simulink model "model"  (R2018a)
settings: Solver=FixedStepAuto  StartTime=0.0  StopTime=inf  FixedStep=0.1  MaxStep=0.1  MinStep=0.001  RelTol=1e-3
libraries: vrlib x19, simulink x15
(part 2 of 2)

== system model/opponent_scout/rand_pos_gen ==
  x_max : Inport
  y_max : Inport  Port=2
  x : Inport  Port=3
  y : Inport  Port=4
  Enable : EnablePort
  Constant : Constant  Value=2
  IC : InitialCondition  Value=0
  Less Than : RelationalOperator  Operator=<  OutDataTypeStr=boolean  RndMeth=Simplest
  Memory : Memory
  Terminator : Terminator
  get_vector : Subsystem
  rand_position_gen : Subsystem
  new_x : Outport
  new_y : Outport  Port=2
  wires:
  get_vector/2(angle) -> Terminator/1
  y/1 -> get_vector/4(y1)
  Less Than/1 -> Memory/1
  Memory/1 -> rand_position_gen/Trigger
  x_max/1 -> rand_position_gen/1(x_max)
  x/1 -> get_vector/2(x1)
  rand_position_gen/1(x_out) -> new_x/1, get_vector/1(x2)
  get_vector/1(distance) -> IC/1
  rand_position_gen/2(y_out) -> new_y/1, get_vector/3(y2)
  y_max/1 -> rand_position_gen/2(y_max)
  Constant/1 -> Less Than/2
  IC/1 -> Less Than/1

== system model/scout/est_theta ==
  r : Inport
  l : Inport  Port=2
  ur : Inport  Port=3
  ul : Inport  Port=4
  theta_0 : Inport  Port=5
  Divide : Product  Inputs=**/
  Integrator : Integrator  InitialConditionSource=external
  Minus : Sum  Inputs=+-
  theta : Outport
  wires:
  theta_0/1 -> Integrator/2
  ur/1 -> Minus/2
  l/1 -> Divide/3
  Minus/1 -> Divide/2
  r/1 -> Divide/1
  ul/1 -> Minus/1
  Integrator/1 -> theta/1
  Divide/1 -> Integrator/1

== system model/scout/est_x ==
  r : Inport
  theta : Inport  Port=2
  ul : Inport  Port=3
  ur : Inport  Port=4
  x0 : Inport  Port=5
  Add : Sum
  Cos : Trigonometry  Operator=cos
  Gain : Gain  Gain=1/2
  Integrator : Integrator  InitialConditionSource=external
  Multiply : Product  Inputs=3
  x : Outport
  wires:
  r/1 -> Multiply/1
  ur/1 -> Add/2
  Add/1 -> Multiply/2
  theta/1 -> Cos/1
  Cos/1 -> Multiply/3
  Integrator/1 -> x/1
  Multiply/1 -> Gain/1
  ul/1 -> Add/1
  Gain/1 -> Integrator/1
  x0/1 -> Integrator/2

== system model/scout/est_y ==
  r : Inport
  theta : Inport  Port=2
  ul : Inport  Port=3
  ur : Inport  Port=4
  y0 : Inport  Port=5
  ref_y : Inport  Port=6
  Add : Sum
  Cos : Trigonometry
  Detect Change : simulink/Logic and Bit Operations/Detect Change  vinit=0  OutDataTypeStr=boolean
  Gain : Gain  Gain=1/2
  Integrator : Integrator  ExternalReset=rising  InitialConditionSource=external
  Multiply : Product  Inputs=3
  Switch : Switch  Criteria=u2 > Threshold
  y : Outport
  wires:
  r/1 -> Multiply/1
  ur/1 -> Add/2
  Add/1 -> Multiply/2
  theta/1 -> Cos/1
  Cos/1 -> Multiply/3
  Integrator/1 -> y/1
  Multiply/1 -> Gain/1
  ul/1 -> Add/1
  Gain/1 -> Integrator/1
  y0/1 -> Switch/3
  ref_y/1 -> Switch/1, Detect Change/1
  Detect Change/1 -> Switch/2, Integrator/2
  Switch/1 -> Integrator/3

== system model/scout/get_vector_to_destination ==
  x2 : Inport
  x1 : Inport  Port=2
  y2 : Inport  Port=3
  y1 : Inport  Port=4
  Add : Sum
  Atan2 : Trigonometry  Operator=atan2
  Minus : Sum  Inputs=+-
  Minus1 : Sum  Inputs=+-
  Sqrt : Sqrt  SaturateOnIntegerOverflow=on
  Square : Math  Operator=square  SaturateOnIntegerOverflow=on
  Square1 : Math  Operator=square  SaturateOnIntegerOverflow=on
  distance : Outport
  angle : Outport  Port=2
  wires:
  Minus/1 -> Atan2/2, Square1/1
  y1/1 -> Minus1/2
  Square/1 -> Add/2
  Minus1/1 -> Atan2/1, Square/1
  Add/1 -> Sqrt/1
  Square1/1 -> Add/1
  x1/1 -> Minus/2
  x2/1 -> Minus/1
  Sqrt/1 -> distance/1
  y2/1 -> Minus1/1
  Atan2/1 -> angle/1

== system model/scout/pid ==
  ref_out : Inport
  act_out : Inport  Port=2
  Kp : Inport  Port=3
  Ki : Inport  Port=4
  Kd : Inport  Port=5
  Enable : EnablePort  StatesWhenEnabling=reset
  Discrete Derivative : simulink/Discrete/Discrete Derivative  gainval=1.0  ICPrevScaledInput=0.0  OutMin=[]  OutMax=[]  OutDataType=fixdt(1, 16)  OutScaling=2^-10  DoSatur=off
  Integrator : Integrator
  Multiply : Product
  Multiply1 : Product
  Multiply2 : Product
  Sum : Sum  Inputs=|+-
  Sum1 : Sum  Inputs=+++
  new_out : Outport
  wires:
  act_out/1 -> Sum/2
  Ki/1 -> Multiply1/2
  Multiply/1 -> Sum1/1
  Kd/1 -> Multiply2/2
  Sum/1 -> Multiply/1, Integrator/1, Discrete Derivative/1
  Kp/1 -> Multiply/2
  ref_out/1 -> Sum/1
  Integrator/1 -> Multiply1/1
  Multiply1/1 -> Sum1/2
  Multiply2/1 -> Sum1/3
  Sum1/1 -> new_out/1
  Discrete Derivative/1 -> Multiply2/1

== system model/scout/pid1 ==
  ref_out : Inport
  act_out : Inport  Port=2
  Kp : Inport  Port=3
  Ki : Inport  Port=4
  Kd : Inport  Port=5
  Enable : EnablePort  StatesWhenEnabling=reset
  Discrete Derivative : simulink/Discrete/Discrete Derivative  gainval=1.0  ICPrevScaledInput=0.0  OutMin=[]  OutMax=[]  OutDataType=fixdt(1, 16)  OutScaling=2^-10  DoSatur=off
  Integrator : Integrator
  Multiply : Product
  Multiply1 : Product
  Multiply2 : Product
  Sum : Sum  Inputs=|+-
  Sum1 : Sum  Inputs=+++
  new_out : Outport
  wires:
  Discrete Derivative/1 -> Multiply2/1
  Sum1/1 -> new_out/1
  Multiply2/1 -> Sum1/3
  Multiply1/1 -> Sum1/2
  Integrator/1 -> Multiply1/1
  ref_out/1 -> Sum/1
  Kp/1 -> Multiply/2
  Sum/1 -> Discrete Derivative/1, Integrator/1, Multiply/1
  Kd/1 -> Multiply2/2
  Multiply/1 -> Sum1/1
  Ki/1 -> Multiply1/2
  act_out/1 -> Sum/2

== system model/scout/rand_pos_gen ==
  x_max : Inport
  y_max : Inport  Port=2
  x : Inport  Port=3
  y : Inport  Port=4
  Constant : Constant  Value=2
  Less Than : RelationalOperator  Operator=<  OutDataTypeStr=boolean  RndMeth=Simplest
  Memory : Memory
  Terminator : Terminator
  get_vector : Subsystem
  rand_position_gen : Subsystem
  new_x : Outport
  new_y : Outport  Port=2
  wires:
  get_vector/2(angle) -> Terminator/1
  y/1 -> get_vector/4(y1)
  Less Than/1 -> Memory/1
  Memory/1 -> rand_position_gen/Trigger
  x_max/1 -> rand_position_gen/1(x_max)
  x/1 -> get_vector/2(x1)
  rand_position_gen/1(x_out) -> new_x/1, get_vector/1(x2)
  get_vector/1(distance) -> Less Than/1
  rand_position_gen/2(y_out) -> new_y/1, get_vector/3(y2)
  y_max/1 -> rand_position_gen/2(y_max)
  Constant/1 -> Less Than/2

== system model/scout/real_theta ==
  r : Inport
  l : Inport  Port=2
  ur : Inport  Port=3
  ul : Inport  Port=4
  theta_0 : Inport  Port=5
  Divide : Product  Inputs=**/
  Integrator : Integrator  InitialConditionSource=external
  Minus : Sum  Inputs=+-
  theta : Outport
  wires:
  theta_0/1 -> Integrator/2
  ur/1 -> Minus/2
  l/1 -> Divide/3
  Minus/1 -> Divide/2
  r/1 -> Divide/1
  ul/1 -> Minus/1
  Integrator/1 -> theta/1
  Divide/1 -> Integrator/1

== system model/scout/real_x ==
  r : Inport
  theta : Inport  Port=2
  ul : Inport  Port=3
  ur : Inport  Port=4
  x0 : Inport  Port=5
  dx_in : Inport  Port=6
  Add : Sum
  Cos : Trigonometry  Operator=cos
  Gain : Gain  Gain=1/2
  Gain1 : Gain  Gain=1.1
  Integrator : Integrator  InitialConditionSource=external
  Multiply : Product  Inputs=3
  Switch : Switch  Criteria=u2 ~= 0
  x : Outport
  dx : Outport  Port=2
  wires:
  r/1 -> Multiply/1
  ur/1 -> Add/2
  Add/1 -> Multiply/2
  theta/1 -> Cos/1
  Cos/1 -> Multiply/3
  Integrator/1 -> x/1
  Multiply/1 -> Gain/1
  ul/1 -> Add/1
  Gain/1 -> Switch/3, dx/1
  x0/1 -> Integrator/2
  dx_in/1 -> Switch/2, Gain1/1
  Switch/1 -> Integrator/1
  Gain1/1 -> Switch/1

== system model/scout/real_y ==
  r : Inport
  theta : Inport  Port=2
  ul : Inport  Port=3
  ur : Inport  Port=4
  y0 : Inport  Port=5
  dy_in : Inport  Port=6
  Add : Sum
  Cos : Trigonometry
  Gain : Gain  Gain=1/2
  Gain1 : Gain  Gain=1.1
  Integrator : Integrator  InitialConditionSource=external
  Multiply : Product  Inputs=3
  Switch : Switch  Criteria=u2 ~= 0
  y : Outport
  dy : Outport  Port=2
  wires:
  r/1 -> Multiply/1
  ur/1 -> Add/2
  Add/1 -> Multiply/2
  theta/1 -> Cos/1
  Cos/1 -> Multiply/3
  Integrator/1 -> y/1
  Multiply/1 -> Gain/1
  ul/1 -> Add/1
  Gain/1 -> Switch/3, dy/1
  y0/1 -> Integrator/2
  dy_in/1 -> Gain1/1, Switch/2
  Switch/1 -> Integrator/1
  Gain1/1 -> Switch/1

== system model/light_spot/rand_pos_gen/get_vector ==
  x2 : Inport
  x1 : Inport  Port=2
  y2 : Inport  Port=3
  y1 : Inport  Port=4
  Add : Sum
  Atan2 : Trigonometry  Operator=atan2
  Minus : Sum  Inputs=+-
  Minus1 : Sum  Inputs=+-
  Sqrt : Sqrt  SaturateOnIntegerOverflow=on
  Square : Math  Operator=square  SaturateOnIntegerOverflow=on
  Square1 : Math  Operator=square  SaturateOnIntegerOverflow=on
  distance : Outport
  angle : Outport  Port=2
  wires:
  Minus/1 -> Atan2/2, Square1/1
  y1/1 -> Minus1/2
  Square/1 -> Add/2
  Minus1/1 -> Atan2/1, Square/1
  Add/1 -> Sqrt/1
  Square1/1 -> Add/1
  x1/1 -> Minus/2
  x2/1 -> Minus/1
  Sqrt/1 -> distance/1
  y2/1 -> Minus1/1
  Atan2/1 -> angle/1

== system model/light_spot/rand_pos_gen/rand_position_gen ==
  x_max : Inport
  y_max : Inport  Port=2
  Trigger : TriggerPort  VariantControl=Variant  PortDimensions=1
  Multiply : Product
  Multiply1 : Product
  x : UniformRandomNumber  Minimum=0  Seed=172
  y : UniformRandomNumber  Minimum=0  Seed=22
  x_out : Outport
  y_out : Outport  Port=2
  wires:
  y_max/1 -> Multiply/1
  x/1 -> Multiply1/2
  y/1 -> Multiply/2
  x_max/1 -> Multiply1/1
  Multiply1/1 -> x_out/1
  Multiply/1 -> y_out/1

== system model/opponent_collector/rand_pos_gen/get_vector ==
  x2 : Inport
  x1 : Inport  Port=2
  y2 : Inport  Port=3
  y1 : Inport  Port=4
  Add : Sum
  Atan2 : Trigonometry  Operator=atan2
  Minus : Sum  Inputs=+-
  Minus1 : Sum  Inputs=+-
  Sqrt : Sqrt  SaturateOnIntegerOverflow=on
  Square : Math  Operator=square  SaturateOnIntegerOverflow=on
  Square1 : Math  Operator=square  SaturateOnIntegerOverflow=on
  distance : Outport
  angle : Outport  Port=2
  wires:
  Minus/1 -> Atan2/2, Square1/1
  y1/1 -> Minus1/2
  Square/1 -> Add/2
  Minus1/1 -> Atan2/1, Square/1
  Add/1 -> Sqrt/1
  Square1/1 -> Add/1
  x1/1 -> Minus/2
  x2/1 -> Minus/1
  Sqrt/1 -> distance/1
  y2/1 -> Minus1/1
  Atan2/1 -> angle/1

== system model/opponent_collector/rand_pos_gen/rand_position_gen ==
  x_max : Inport
  y_max : Inport  Port=2
  Trigger : TriggerPort  VariantControl=Variant  PortDimensions=1
  Multiply : Product
  Multiply1 : Product
  x : UniformRandomNumber  Minimum=0  Seed=1
  y : UniformRandomNumber  Minimum=0  Seed=110
  x_out : Outport
  y_out : Outport  Port=2
  wires:
  y_max/1 -> Multiply/1
  x/1 -> Multiply1/2
  y/1 -> Multiply/2
  x_max/1 -> Multiply1/1
  Multiply1/1 -> x_out/1
  Multiply/1 -> y_out/1

== system model/opponent_scout/rand_pos_gen/get_vector ==
  x2 : Inport
  x1 : Inport  Port=2
  y2 : Inport  Port=3
  y1 : Inport  Port=4
  Add : Sum
  Atan2 : Trigonometry  Operator=atan2
  Minus : Sum  Inputs=+-
  Minus1 : Sum  Inputs=+-
  Sqrt : Sqrt  SaturateOnIntegerOverflow=on
  Square : Math  Operator=square  SaturateOnIntegerOverflow=on
  Square1 : Math  Operator=square  SaturateOnIntegerOverflow=on
  distance : Outport
  angle : Outport  Port=2
  wires:
  Minus/1 -> Atan2/2, Square1/1
  y1/1 -> Minus1/2
  Square/1 -> Add/2
  Minus1/1 -> Atan2/1, Square/1
  Add/1 -> Sqrt/1
  Square1/1 -> Add/1
  x1/1 -> Minus/2
  x2/1 -> Minus/1
  Sqrt/1 -> distance/1
  y2/1 -> Minus1/1
  Atan2/1 -> angle/1

== system model/opponent_scout/rand_pos_gen/rand_position_gen ==
  x_max : Inport
  y_max : Inport  Port=2
  Trigger : TriggerPort  VariantControl=Variant  PortDimensions=1
  Multiply : Product
  Multiply1 : Product
  x : UniformRandomNumber  Minimum=0  Seed=213
  y : UniformRandomNumber  Minimum=0  Seed=130
  x_out : Outport
  y_out : Outport  Port=2
  wires:
  y_max/1 -> Multiply/1
  x/1 -> Multiply1/2
  y/1 -> Multiply/2
  x_max/1 -> Multiply1/1
  Multiply1/1 -> x_out/1
  Multiply/1 -> y_out/1

== system model/scout/rand_pos_gen/get_vector ==
  x2 : Inport
  x1 : Inport  Port=2
  y2 : Inport  Port=3
  y1 : Inport  Port=4
  Add : Sum
  Atan2 : Trigonometry  Operator=atan2
  Minus : Sum  Inputs=+-
  Minus1 : Sum  Inputs=+-
  Sqrt : Sqrt  SaturateOnIntegerOverflow=on
  Square : Math  Operator=square  SaturateOnIntegerOverflow=on
  Square1 : Math  Operator=square  SaturateOnIntegerOverflow=on
  distance : Outport
  angle : Outport  Port=2
  wires:
  Minus/1 -> Atan2/2, Square1/1
  y1/1 -> Minus1/2
  Square/1 -> Add/2
  Minus1/1 -> Atan2/1, Square/1
  Add/1 -> Sqrt/1
  Square1/1 -> Add/1
  x1/1 -> Minus/2
  x2/1 -> Minus/1
  Sqrt/1 -> distance/1
  y2/1 -> Minus1/1
  Atan2/1 -> angle/1

== system model/scout/rand_pos_gen/rand_position_gen ==
  x_max : Inport
  y_max : Inport  Port=2
  Trigger : TriggerPort  VariantControl=Variant  PortDimensions=1
  Multiply : Product
  Multiply1 : Product
  x : UniformRandomNumber  Minimum=0  Seed=56
  y : UniformRandomNumber  Minimum=0  Seed=87
  x_out : Outport
  y_out : Outport  Port=2
  wires:
  y_max/1 -> Multiply/1
  x/1 -> Multiply1/2
  y/1 -> Multiply/2
  x_max/1 -> Multiply1/1
  Multiply1/1 -> x_out/1
  Multiply/1 -> y_out/1

== matlab function model/scout_receiver/scout_receiver ==
  data: clk input; out_of_bounds output; byte input; x output; y output; theta output
function [out_of_bounds,x,y,theta] = fcn(clk, byte)
out_of_bounds = 0;
x = 255;
y = 255;
theta = 255;
if byte == hex2dec('31')
    out_of_bounds = 1;
elseif mod(clk,10) <= 0.3
elseif mod(clk,10) <= 0.6
    x = byte * 2;
elseif mod(clk,10) <= 0.9
    y = byte * 2;
elseif mod(clk,10) <= 1.2
    theta = byte * 2 / 180 * pi;
end
end

== matlab function model/referee/transmitter ==
  data: clk input; scout_x input; byte output; scout_y input; scout_th input; coll_x input; coll_y input; coll_th input; x_max input; y_max input
function byte = fcn(clk, scout_x, scout_y, scout_th, coll_x, coll_y, coll_th, x_max, y_max)

if mod(clk,10) <= 0.3
    byte = hex2dec('21');
elseif mod(clk,10) <= 0.6
    byte = scout_x;
elseif mod(clk,10) <= 0.9
    byte = scout_y;
elseif mod(clk,10) <= 1.2
    byte = scout_th;
elseif mod(clk,10) <= 1.5
    byte = hex2dec('22');
elseif mod(clk,10) <= 1.8
    byte = coll_x;
elseif mod(clk,10) <= 2.1
    byte = coll_y;
elseif mod(clk,10) <= 2.4
    byte = coll_th;
elseif scout_x > x_max || scout_x < 0 || scout_y > y_max || scout_y < 0
    byte = hex2dec('31');
elseif coll_x > x_max || coll_x < 0 || coll_y > y_max || coll_y < 0
    byte = hex2dec('32');
else
    byte = 0;
end
end

== matlab function model/collector_receiver/collector_receiver ==
  data: clk input; out_of_bounds output; byte input; x output; y output; theta output
function [out_of_bounds,x,y,theta] = fcn(clk, byte)
out_of_bounds = 0;
x = 255;
y = 255;
theta = 255;
if byte == hex2dec('32')
    out_of_bounds = 1;
elseif mod(clk,10) <= 1.5
elseif mod(clk,10) <= 1.8
    x = byte * 2;
elseif mod(clk,10) <= 2.1
    y = byte * 2;
elseif mod(clk,10) <= 2.4
    theta = byte * 2 / 180 * pi;    
end
end

== matlab function model/MATLAB Function ==
  data: u input; sc_opsc output; col_opsc output; opcol_opsc output; opsc_sc output; col_sc output; opcol_sc output; opsc_col output; sc_col output; opcol_col output; opsc_opcol output; sc_opcol output; col_opcol output
function [sc_opsc,col_opsc,opcol_opsc,opsc_sc,col_sc,opcol_sc,opsc_col,sc_col,opcol_col,opsc_opcol,sc_opcol,col_opcol] = fcn(u)
sc_opsc = u(2,1);
col_opsc = u(3,1);
opcol_opsc = u(4,1);
opsc_sc = u(1,2);
col_sc = u(3,2);
opcol_sc = u(4,2);
opsc_col = u(1,3);
sc_col = u(2,3);
opcol_col = u(4,3);
opsc_opcol = u(1,4);
sc_opcol = u(2,4);
col_opcol = u(3,4);
